simulink library "sim_stud_lib_r2022a"  (R2022a)
settings: Solver=VariableStepAuto  StartTime=0.0  StopTime=10.0  RelTol=1e-3
settings Model: Creator=iVBk  LastModifiedBy=RolePups
settings ModelReferenceCC: EnableRefExpFcnMdlSchedulingChecks=off
settings RTWCC: Description=Generic Real-Time Target

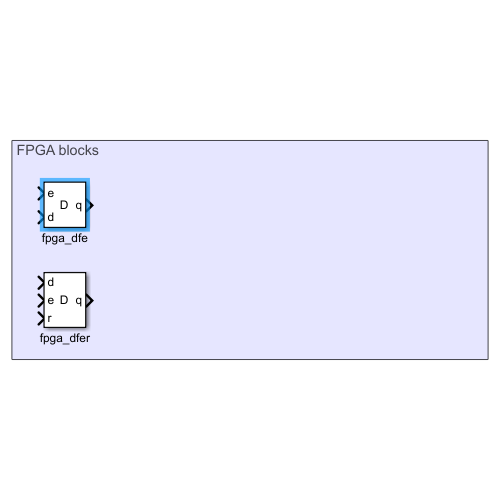
[thumbnail: Simulink's stored preview of the top-level diagram]
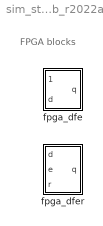
== system sim_stud_lib_r2022a ==
  note: FPGA blocks
  fpga_dfe : Subsystem
      mask Display:
      | disp('D');
      | port_label('input',1,'e');
      | port_label('input',2,'d');
      | port_label('output',1,'q');
  fpga_dfer : Subsystem
      mask Display:
      | disp('D');
      | port_label('input',1,'d');
      | port_label('input',2,'e');
      | port_label('input',3,'r');
      | port_label('output',1,'q');

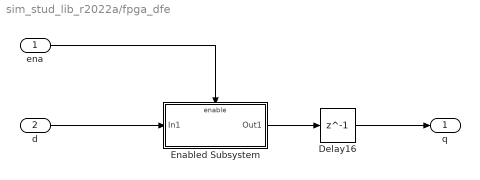
== system sim_stud_lib_r2022a/fpga_dfe ==
  ena : Inport
  d : Inport  Port=2
  Delay16 : Delay  DelayLength=1
  Enabled Subsystem : Subsystem  TreatAsAtomicUnit=on
  q : Outport  VectorParamsAs1DForOutWhenUnconnected=off
  wires:
  d/1 -> Enabled Subsystem/1(In1)
  ena/1 -> Enabled Subsystem/Enable
  Delay16/1 -> q/1
  Enabled Subsystem/1(Out1) -> Delay16/1

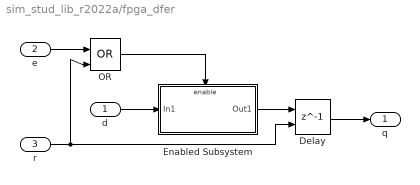
== system sim_stud_lib_r2022a/fpga_dfer ==
  d : Inport
  e : Inport  Port=2
  r : Inport  Port=3
  Delay : Delay  DelayLength=1  ExternalReset=Level hold
      settings: InputPortMap=u0,r5
  Enabled Subsystem : Subsystem  TreatAsAtomicUnit=on
  OR : Logic  Operator=OR  IconShape=distinctive  AllPortsSameDT=off  OutDataTypeStr=boolean
  q : Outport
  wires:
  r/1 -> Delay/2, OR/2
  e/1 -> OR/1
  OR/1 -> Enabled Subsystem/Enable
  Delay/1 -> q/1
  Enabled Subsystem/1(Out1) -> Delay/1
  d/1 -> Enabled Subsystem/1(In1)

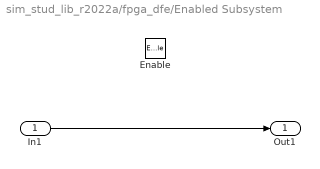
== system sim_stud_lib_r2022a/fpga_dfe/Enabled Subsystem ==
  In1 : Inport
  Enable : EnablePort
  Out1 : Outport  VectorParamsAs1DForOutWhenUnconnected=off
  wires:
  In1/1 -> Out1/1

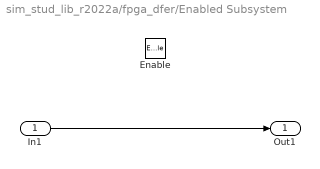
== system sim_stud_lib_r2022a/fpga_dfer/Enabled Subsystem ==
  In1 : Inport
  Enable : EnablePort
  Out1 : Outport
  wires:
  In1/1 -> Out1/1
